simulink subsystem "Make_Knots"  (R2023b)
settings: Solver=VariableStepAuto  StartTime=0.0  StopTime=10.0  RelTol=1e-3
undefined symbols (not defined in the file): Spline_Max_Num_RefPoses
libraries: simulink x1
settings Model: Creator=FIRSTMentor  LastModifiedBy=ander

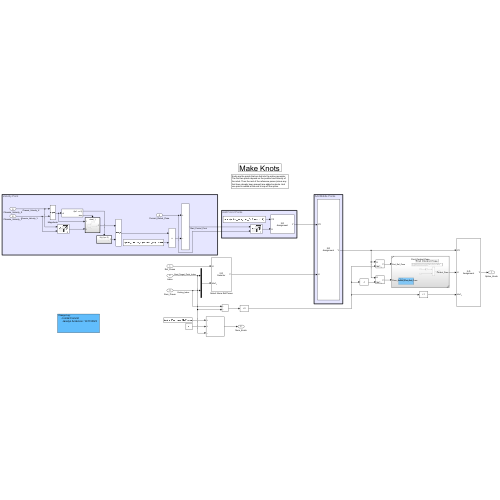
[thumbnail: Simulink's stored preview of the top-level diagram]
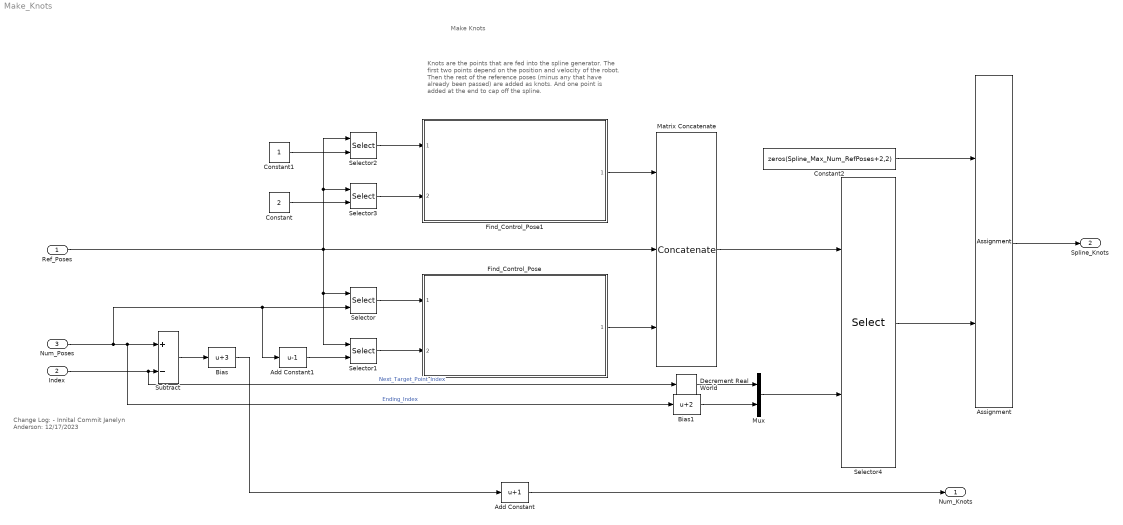
== system Make_Knots ==
  note: Knots are the points that are fed into the spline generator. The first two points depend on the position and velocity of the robot. Then the rest of the reference poses (minus any that have already been passed) are added as knots. And one point is added at the end to cap off the spline.
  note: Make Knots
  note: Change Log:
      | - Innital Commit
      | Janelyn Anderson: 12/17/2023
  Ref_Poses : Inport
  Index : Inport  Port=2
  Num_Poses : Inport  Port=3
  Add Constant : Bias  Bias=1  SaturateOnIntegerOverflow=off
  Add Constant1 : Bias  Bias=-1  SaturateOnIntegerOverflow=off
  Assignment : Assignment  NumberOfDimensions=2  DiagnosticForDimensions=Warning  IndexOptions=Starting index (dialog),Assign all  Indices=1,1  OutputSizes=1,1
  Bias : Bias  Bias=3  SaturateOnIntegerOverflow=off
  Bias1 : Bias  Bias=2  SaturateOnIntegerOverflow=off
  Constant : Constant  Value=2
  Constant1 : Constant
  Constant2 : Constant  Value=zeros(Spline_Max_Num_RefPoses+2,2)
  Decrement Real World : simulink/Additional Math & Discrete/Additional Math: Increment - Decrement/Decrement Real World
  Find_Control_Pose : Subsystem  ReferencedSubsystem=Find_Control_Pose
  Find_Control_Pose1 : Subsystem  ReferencedSubsystem=Find_Control_Pose
  Matrix Concatenate : Concatenate  NumInputs=3  Mode=Multidimensional array
  Mux : Mux  Inputs=2
  Selector{,1..3} (4 alike) : Selector  NumberOfDimensions=2  InputPortWidth=3  IndexOptions=Index vector (port),Select all  Indices=[1 3],1  OutputSizes=1,1
  Selector4 : Selector  NumberOfDimensions=2  InputPortWidth=3  IndexOptions=Starting and ending indices (port),Select all  Indices=[1 3],1  OutputSizes=1,1
  Subtract : Sum  Inputs=+-
  Num_Knots : Outport
  Spline_Knots : Outport  Port=2
  wires:
  Bias/1 -> Add Constant/1
  Ref_Poses/1 -> Matrix Concatenate/2, Selector2/1, Selector3/1, Selector/1, Selector1/1
  Add Constant1/1 -> Selector1/2
  Selector1/1 -> Find_Control_Pose/2
  Matrix Concatenate/1 -> Selector4/1
  Subtract/1 -> Bias/1
  Selector/1 -> Find_Control_Pose/1
  Num_Poses/1 -> Selector/2, Add Constant1/1, Subtract/1, Bias1/1  "Ending_Index"
  Index/1 -> Subtract/2, Decrement Real World/1  "Next_Target_Point_Index"
  Add Constant/1 -> Num_Knots/1
  Find_Control_Pose/1 -> Matrix Concatenate/3
  Find_Control_Pose1/1 -> Matrix Concatenate/1
  Selector3/1 -> Find_Control_Pose1/2
  Selector2/1 -> Find_Control_Pose1/1
  Constant1/1 -> Selector2/2
  Constant/1 -> Selector3/2
  Selector4/1 -> Assignment/2
  Mux/1 -> Selector4/2
  Decrement Real World/1 -> Mux/1
  Bias1/1 -> Mux/2
  Constant2/1 -> Assignment/1
  Assignment/1 -> Spline_Knots/1
